simulink model "SimpleGrid"  (R2020b)
settings: Solver=ode45  StartTime=0.0  StopTime=100  MaxStep=1e-4  RelTol=1e-4  EnableMultiTasking=on
libraries: powerlib_meascontrol x4, powerlib x1
settings Model: Creator=edu  LastModifiedBy=eprie
settings DataIOCC: LimitDataPoints=on  SaveFormat=Array  SignalLoggingSaveFormat=ModelDataLogs  ReturnWorkspaceOutputs=off
settings OptimizationCC: ExpressionDepthLimit=2147483647  LifeSpan=inf
settings DebuggingCC: UnderspecifiedInitializationDetection=Classic  MergeDetectMultiDrivingBlocksExec=none  SolverPrmCheckMsg=warning  FcnCallInpInsideContextMsg=warning  AllowSymbolicDim=off  StateNameClashWarn=warning  SFUnexpectedBacktrackingDiag=warning  SFNoUnconditionalDefaultTransitionDiag=warning  SFExecutionAtInitializationDiag=none  ArithmeticOperatorsInVariantConditions=warning
settings HardwareCC: ProdBitPerPointer=32  ProdBitPerSizeT=32  ProdBitPerPtrDiffT=32  ProdLargestAtomicFloat=None  ProdIntDivRoundTo=Undefined  ProdEndianess=Unspecified  ProdWordSize=32  ProdHWDeviceType=32-bit Generic
settings ModelReferenceCC: PropagateSignalLabelsOutOfModel=off
settings SFSimCC: SimUseLocalCustomCode=off  CustomCodeUndefinedFunction=UseInterfaceOnly
settings RTWCC: RTWUseLocalCustomCode=off
settings CodeAppCC: StateflowObjectComments=on
settings GRTTargetCC: TargetLangStandard=C89/C90 (ANSI)  CombineOutputUpdateFcns=off  GRTInterface=on
settings ConfigComp: CovMetricSettings=dw  CovSaveCumulativeToWorkspaceVar=on  CovSaveSingleToWorkspaceVar=on  CovExternalEMLEnable=off
settings SimscapeCC: SimscapeNormalizeSystem=off
settings ConfigurationSet: Description=SimMechanics 2G

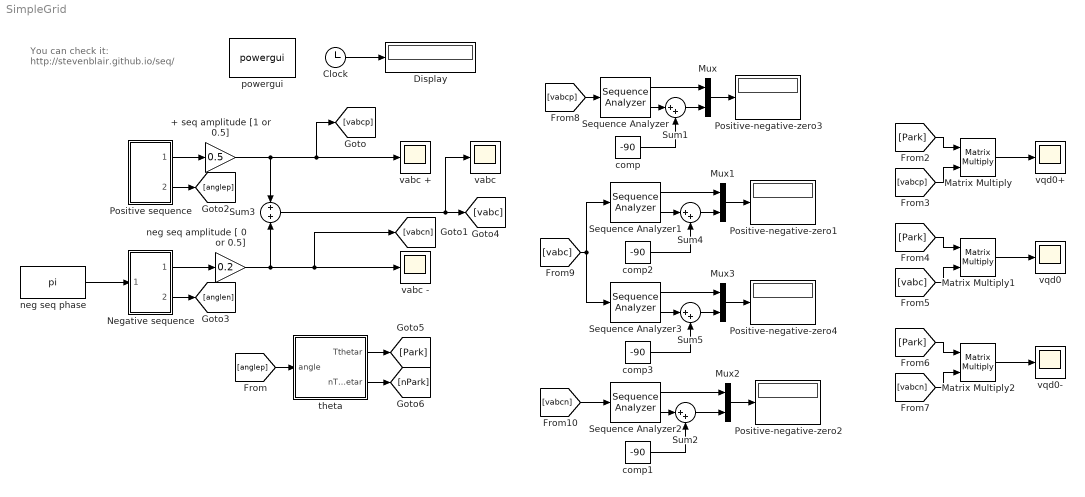
== system SimpleGrid ==
  note: You can check it:
      | http://stevenblair.github.io/seq/
  + seq amplitude [1 or 0.5] : Gain  Gain=0.5
  Clock : Clock
  Display : Display
  Matrix Multiply : Product  Multiplication=Matrix(*)
  Matrix Multiply1 : Product  Multiplication=Matrix(*)
  Matrix Multiply2 : Product  Multiplication=Matrix(*)
  Mux{,1..3} (4 alike) : Mux  Inputs=2
  Negative sequence : Subsystem
  Positive sequence : Subsystem
  Positive-negative-zero{1..4} (4 alike) : Display
  Sequence Analyzer : powerlib_meascontrol/Measurements/Sequence Analyzer  Freq=50  n=1  seq=Positive  InInit=[1, 0]  Ts=0
      settings: SourceProductBaseCode=PS
  Sequence Analyzer1 : powerlib_meascontrol/Measurements/Sequence Analyzer  Freq=50  n=1  seq=Positive  InInit=[1, 0]  Ts=0
      settings: SourceProductBaseCode=PS
  Sequence Analyzer2 : powerlib_meascontrol/Measurements/Sequence Analyzer  Freq=50  n=1  seq=Negative  InInit=[1, 0]  Ts=0
      settings: SourceProductBaseCode=PS
  Sequence Analyzer3 : powerlib_meascontrol/Measurements/Sequence Analyzer  Freq=50  n=1  seq=Negative  InInit=[1, 0]  Ts=0
      settings: SourceProductBaseCode=PS
  Sum{1..2,4..5} (4 alike) : Sum  Inputs=|++
  Sum3 : Sum
  comp{,1..3} (4 alike) : Constant  Value=-90
  neg seq amplitude [ 0 or 0.5] : Gain  Gain=0.2
  neg seq phase : Constant  Value=pi
  powergui : powerlib/powergui  Priority=1  SimulationMode=Continuous  SampleTime=50e-6  frequency=60  Iterations=50  frequencyindice=0  Pbase=100e6  ErrMax=1e-4  UnitsV=kV  UnitsW=MW  buscounter=0  FunctionMessages=off  echomessages=off  EnableUseOfTLC=off  CurrentSourceSwitches=off  DisableSnubberDevices=off  DisableRonSwitches=off  DisableVfSwitches=off  DisplayEquations=off  AutomaticDiscreteSolvers=off  SolverType=Tustin  Interpol=off  ExternalGateDelay=off  methode=off  Ts=10  x0status=blocks  SPID=off  SwTol=0  HookPort=off  NonlinearTolerance=1e-4  nMaxIteration=100  ContinueOnMaxIteration=off  RestoreLinks=warning  ResistiveCurrentMeasurement=off  Frange=[0:2:500]  Ylog=off  Xlog=on  ShowGrid=off  save=off  variable=ZData  structure=0  ZoomFFT=off  StartTime=0.0  cycles=1  DisplayStyle=1  fundamental=60  FreqAxis=off  MaxFrequency=1000  frequencyindicesteady=1  RmsSteady=1  display=off
  theta : Subsystem
  vabc : Scope
  vabc + : Scope
  vabc - : Scope
  vqd0 : Scope
  vqd0+ : Scope
  vqd0- : Scope
  wires:
  Clock/1 -> Display/1
  Positive sequence/1(vabc +) -> + seq amplitude [1 or 0.5]/1
  Negative sequence/1(vabc -) -> neg seq amplitude [ 0 or 0.5]/1
  neg seq amplitude [ 0 or 0.5]/1 -> [vabcn], vabc -/1, Sum3/2
  Positive sequence/2(angle +) -> [anglep]
  Negative sequence/2(angle -) -> [anglen]
  [anglep] -> theta/1(angle)
  Sum3/1 -> vabc/1, [vabc]
  theta/1(Tthetar) -> [Park]
  theta/2(nTthetar) -> [nPark]
  [Park] -> Matrix Multiply/1
  [vabcp] -> Matrix Multiply/2
  [Park] -> Matrix Multiply1/1
  [vabc] -> Matrix Multiply1/2
  [Park] -> Matrix Multiply2/1
  [vabcn] -> Matrix Multiply2/2
  Matrix Multiply/1 -> vqd0+/1
  Matrix Multiply1/1 -> vqd0/1
  Matrix Multiply2/1 -> vqd0-/1
  + seq amplitude [1 or 0.5]/1 -> Sum3/1, [vabcp], vabc +/1
  neg seq phase/1 -> Negative sequence/1(phase)
  Sequence Analyzer/1 -> Mux/1
  Mux/1 -> Positive-negative-zero3/1
  Sequence Analyzer1/1 -> Mux1/1
  [vabcp] -> Sequence Analyzer/1
  [vabc] -> Sequence Analyzer1/1, Sequence Analyzer3/1
  [vabcn] -> Sequence Analyzer2/1
  Sequence Analyzer/2 -> Sum1/1
  Sequence Analyzer1/2 -> Sum4/1
  Sum1/1 -> Mux/2
  comp/1 -> Sum1/2
  comp2/1 -> Sum4/2
  Sum4/1 -> Mux1/2
  Mux1/1 -> Positive-negative-zero1/1
  Sequence Analyzer3/1 -> Mux3/1
  Sequence Analyzer3/2 -> Sum5/1
  comp3/1 -> Sum5/2
  Sum5/1 -> Mux3/2
  Mux3/1 -> Positive-negative-zero4/1
  Sequence Analyzer2/1 -> Mux2/1
  Sequence Analyzer2/2 -> Sum2/1
  comp1/1 -> Sum2/2
  Sum2/1 -> Mux2/2
  Mux2/1 -> Positive-negative-zero2/1

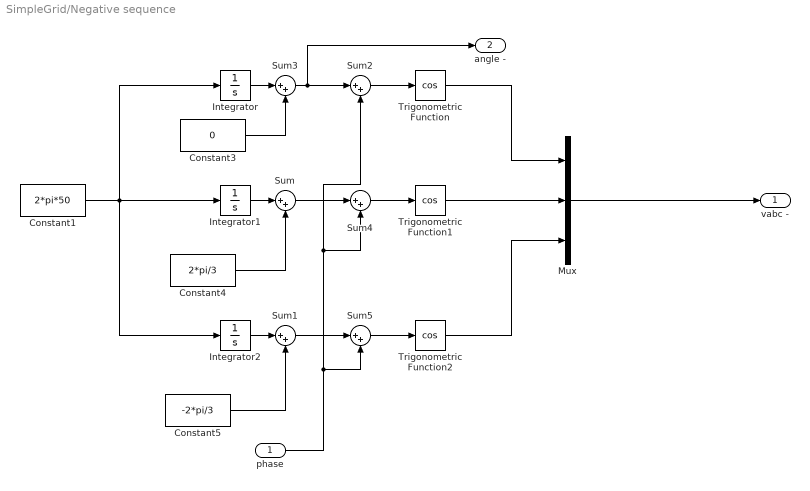
== system SimpleGrid/Negative sequence ==
  phase : Inport
  Constant1 : Constant  Value=2*pi*50
  Constant3 : Constant  Value=0
  Constant4 : Constant  Value=2*pi/3
  Constant5 : Constant  Value=-2*pi/3
  Integrator : Integrator
  Integrator1 : Integrator
  Integrator2 : Integrator
  Mux : Mux  Inputs=3
  Sum{,1..5} (6 alike) : Sum  Inputs=|++
  Trigonometric Function : Trigonometry  Operator=cos
  Trigonometric Function1 : Trigonometry  Operator=cos
  Trigonometric Function2 : Trigonometry  Operator=cos
  vabc - : Outport
  angle - : Outport  Port=2
  wires:
  Integrator/1 -> Sum3/1
  Constant5/1 -> Sum1/2
  Constant1/1 -> Integrator1/1, Integrator/1, Integrator2/1
  Mux/1 -> vabc -/1
  Trigonometric Function1/1 -> Mux/2
  Integrator1/1 -> Sum/1
  Trigonometric Function2/1 -> Mux/3
  Sum3/1 -> angle -/1, Sum2/1
  Constant4/1 -> Sum/2
  Constant3/1 -> Sum3/2
  Integrator2/1 -> Sum1/1
  Trigonometric Function/1 -> Mux/1
  Sum2/1 -> Trigonometric Function/1
  Sum/1 -> Sum4/1
  Sum4/1 -> Trigonometric Function1/1
  Sum1/1 -> Sum5/1
  Sum5/1 -> Trigonometric Function2/1
  phase/1 -> Sum5/2, Sum4/2, Sum2/2

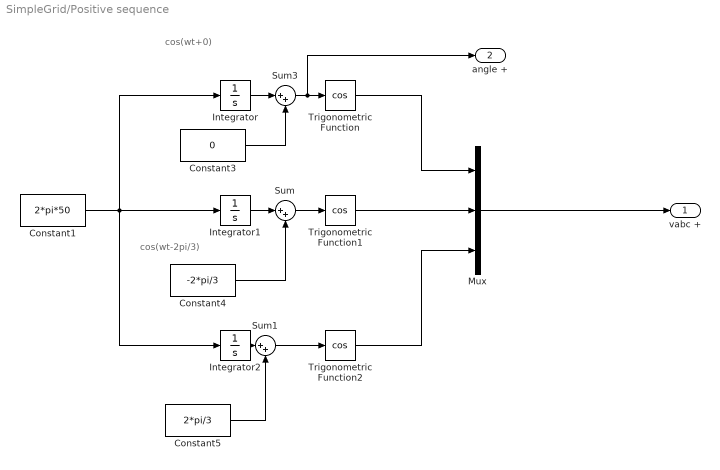
== system SimpleGrid/Positive sequence ==
  note: cos(wt+0)
  note: cos(wt-2pi/3)
  Constant1 : Constant  Value=2*pi*50
  Constant3 : Constant  Value=0
  Constant4 : Constant  Value=-2*pi/3
  Constant5 : Constant  Value=2*pi/3
  Integrator : Integrator
  Integrator1 : Integrator
  Integrator2 : Integrator
  Mux : Mux  Inputs=3
  Sum : Sum  Inputs=|++
  Sum1 : Sum  Inputs=|++
  Sum3 : Sum  Inputs=|++
  Trigonometric Function : Trigonometry  Operator=cos
  Trigonometric Function1 : Trigonometry  Operator=cos
  Trigonometric Function2 : Trigonometry  Operator=cos
  vabc + : Outport
  angle + : Outport  Port=2
  wires:
  Trigonometric Function/1 -> Mux/1
  Sum/1 -> Trigonometric Function1/1
  Integrator2/1 -> Sum1/1
  Constant3/1 -> Sum3/2
  Constant4/1 -> Sum/2
  Sum3/1 -> angle +/1, Trigonometric Function/1
  Trigonometric Function2/1 -> Mux/3
  Integrator1/1 -> Sum/1
  Trigonometric Function1/1 -> Mux/2
  Sum1/1 -> Trigonometric Function2/1
  Mux/1 -> vabc +/1
  Constant1/1 -> Integrator2/1, Integrator/1, Integrator1/1
  Constant5/1 -> Sum1/2
  Integrator/1 -> Sum3/1

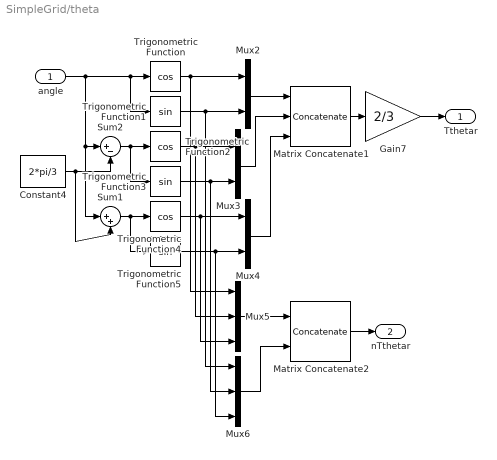
== system SimpleGrid/theta ==
  angle : Inport
  Constant4 : Constant  Value=2*pi/3  SampleTime=0
  Gain7 : Gain  Gain=2/3
  Matrix Concatenate1 : Concatenate  NumInputs=3  Mode=Multidimensional array  ConcatenateDimension=2
  Matrix Concatenate2 : Concatenate  Mode=Multidimensional array  ConcatenateDimension=2
  Mux2 : Mux  Inputs=2
  Mux3 : Mux  Inputs=2
  Mux4 : Mux  Inputs=2
  Mux5 : Mux  Inputs=3
  Mux6 : Mux  Inputs=3
  Sum1 : Sum  Inputs=|++
  Sum2 : Sum  Inputs=|+-
  Trigonometric Function : Trigonometry  Operator=cos
  Trigonometric Function1 : Trigonometry
  Trigonometric Function2 : Trigonometry  Operator=cos
  Trigonometric Function3 : Trigonometry
  Trigonometric Function4 : Trigonometry  Operator=cos
  Trigonometric Function5 : Trigonometry
  Tthetar : Outport
  nTthetar : Outport  Port=2
  wires:
  Matrix Concatenate2/1 -> nTthetar/1
  Gain7/1 -> Tthetar/1
  angle/1 -> Trigonometric Function1/1, Trigonometric Function/1, Sum2/1, Sum1/1
  Mux6/1 -> Matrix Concatenate2/2
  Mux5/1 -> Matrix Concatenate2/1
  Matrix Concatenate1/1 -> Gain7/1
  Mux4/1 -> Matrix Concatenate1/3
  Mux3/1 -> Matrix Concatenate1/2
  Mux2/1 -> Matrix Concatenate1/1
  Trigonometric Function5/1 -> Mux6/3, Mux4/2
  Trigonometric Function4/1 -> Mux5/3, Mux4/1
  Trigonometric Function3/1 -> Mux6/2, Mux3/2
  Trigonometric Function2/1 -> Mux5/2, Mux3/1
  Trigonometric Function1/1 -> Mux6/1, Mux2/2
  Trigonometric Function/1 -> Mux5/1, Mux2/1
  Constant4/1 -> Sum1/2, Sum2/2
  Sum1/1 -> Trigonometric Function5/1, Trigonometric Function4/1
  Sum2/1 -> Trigonometric Function3/1, Trigonometric Function2/1
